simulink model "om1"  (Simulink 7.0)
settings: Solver=ode45  StartTime=0.0  StopTime=10.0  RelTol=1e-3
libraries: cdsFilt x105, cdsIPC x13, cdsEpicsOut x13, cdsMatrix x9, cdsEpicsIn x6, cdsOsc x5, cdsPhase x5, cdsProduct x4, cdsBitwise x4, cdsRms x3, cdsFiltCtrl x2, cdsRfmIO x1
(part 1 of 5)
settings Model: Creator=Rolf  LastModifiedBy=controls  ExtModeAutoUpdateStatusClock=off

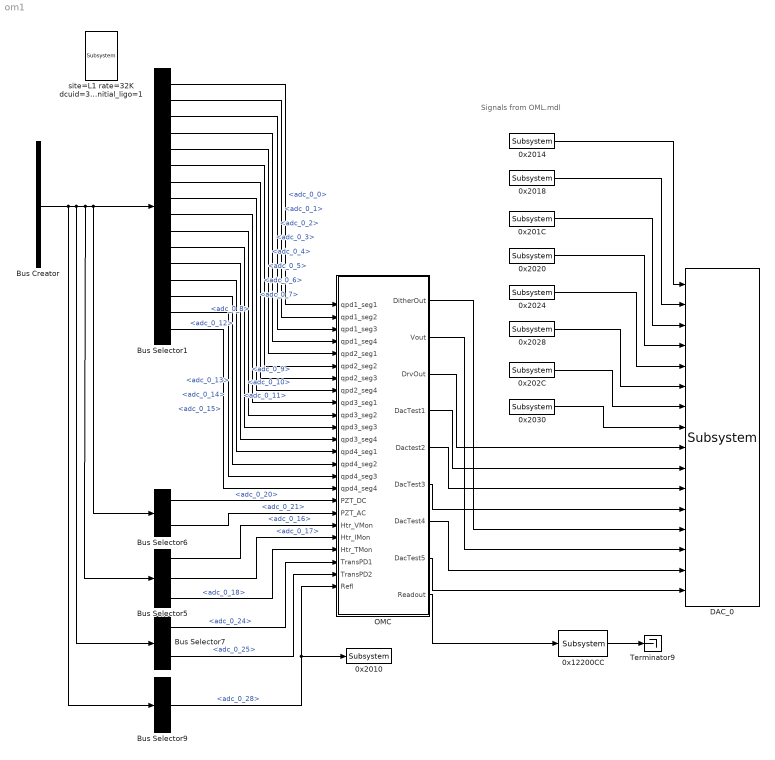
== system om1 ==
  note: Signals from OML.mdl
  0x12200CC : cdsRfmIO/Subsystem  Tag=cdsRfmIO  Description=VMIC5565 Reflective Memory read/write  SystemSampleTime=-1
      settings: AttributesFormatString=%<Tag>
  0x{2010,2014,2018,2020,2024,2028,2030} (7 alike) : cdsIPC/Subsystem  Tag=cdsIPC  Description=Inter-process communication through /rtl_epics_ipc shared memory  SystemSampleTime=-1
      settings: AttributesFormatString=%<Tag>
  0x201C : cdsIPC/Subsystem  Tag=cdsIPC  Description=Inter-process communication through /rtl_epics_ipc shared memory  SystemSampleTime=-1
      settings: AttributesFormatString=%<Tag>
  0x202C : cdsIPC/Subsystem  Tag=cdsIPC  Description=Inter-process communication through /rtl_epics_ipc shared memory  SystemSampleTime=-1
      settings: AttributesFormatString=%<Tag>
  Bus Creator : BusCreator  Tag=adc_0  Description=|  Inputs='adc_0_0','adc_0_1','adc_0_2','adc_0_3','adc_0_4','adc_0_5','adc_0_6','adc_0_7','adc_0_8','adc_0_9','adc_0_10','adc_0_11','adc_0_12','adc_0_13','adc_0_14','adc_0_15','adc_0_16','adc_0_17','adc_0_18','adc_0_19','adc_0_20','adc_0_21','adc_0_22','adc_0_23','adc_0_24','adc_0_25','adc_0_26','adc_0_27','adc_0_28','adc_0_29','adc_0_30','adc_0_31'
      | PCI66-16AI64SSA            
      | 40Vp-p, 16-bit, 610uV/count
      | card_num=1
      settings: AttributesFormatString=%<Description>\n%<Tag>
  Bus Selector1 : BusSelector  OutputSignals=adc_0_0,adc_0_1,adc_0_2,adc_0_3,adc_0_4,adc_0_5,adc_0_6,adc_0_7,adc_0_8,adc_0_9,adc_0_10,adc_0_11,adc_0_12,adc_0_13,adc_0_14,adc_0_15
  Bus Selector5 : BusSelector  OutputSignals=adc_0_16,adc_0_17,adc_0_18
  Bus Selector6 : BusSelector  OutputSignals=adc_0_20,adc_0_21
  Bus Selector7 : BusSelector  OutputSignals=adc_0_24,adc_0_25
  Bus Selector9 : BusSelector  OutputSignals=adc_0_28
  DAC_0 : dac/Subsystem  Description=|  SystemSampleTime=-1
      | PCI66-16AO16
      | 20Vp-p, 16-bit, 305uV/count
      settings: AttributesFormatString=%<Description>
  OMC : Subsystem  Tag=top_names
      settings: AttributesFormatString=%<Tag>
  Terminator9 : Terminator
  site=L1 rate=32K dcuid=30 gds_node_id=4 no_sync=1 compat_initial_ligo=1 : cdsParameters/Subsystem  Tag=cdsParameters  SystemSampleTime=-1
      settings: AttributesFormatString=%<Tag>
  wires:
  Bus Creator/1 -> Bus Selector5/1, Bus Selector1/1, Bus Selector6/1, Bus Selector7/1, Bus Selector9/1
  Bus Selector6/1 -> OMC/17(PZT_DC)  "<adc_0_20>"
  Bus Selector6/2 -> OMC/18(PZT_AC)  "<adc_0_21>"
  Bus Selector7/1 -> OMC/22(TransPD1)  "<adc_0_24>"
  Bus Selector7/2 -> OMC/23(TransPD2)  "<adc_0_25>"
  Bus Selector9/1 -> OMC/24(Refl), 0x2010/1  "<adc_0_28>"
  Bus Selector5/1 -> OMC/19(Htr_VMon)  "<adc_0_16>"
  Bus Selector5/2 -> OMC/20(Htr_IMon)  "<adc_0_17>"
  Bus Selector5/3 -> OMC/21(Htr_TMon)  "<adc_0_18>"
  Bus Selector1/1 -> OMC/1(qpd1_seg1)  "<adc_0_0>"
  Bus Selector1/2 -> OMC/2(qpd1_seg2)  "<adc_0_1>"
  Bus Selector1/3 -> OMC/3(qpd1_seg3)  "<adc_0_2>"
  Bus Selector1/4 -> OMC/4(qpd1_seg4)  "<adc_0_3>"
  Bus Selector1/9 -> OMC/9(qpd3_seg1)  "<adc_0_8>"
  Bus Selector1/10 -> OMC/10(qpd3_seg2)  "<adc_0_9>"
  Bus Selector1/11 -> OMC/11(qpd3_seg3)  "<adc_0_10>"
  Bus Selector1/12 -> OMC/12(qpd3_seg4)  "<adc_0_11>"
  Bus Selector1/5 -> OMC/5(qpd2_seg1)  "<adc_0_4>"
  Bus Selector1/6 -> OMC/6(qpd2_seg2)  "<adc_0_5>"
  Bus Selector1/7 -> OMC/7(qpd2_seg3)  "<adc_0_6>"
  Bus Selector1/8 -> OMC/8(qpd2_seg4)  "<adc_0_7>"
  Bus Selector1/13 -> OMC/13(qpd4_seg1)  "<adc_0_12>"
  Bus Selector1/14 -> OMC/14(qpd4_seg2)  "<adc_0_13>"
  Bus Selector1/15 -> OMC/15(qpd4_seg3)  "<adc_0_14>"
  Bus Selector1/16 -> OMC/16(qpd4_seg4)  "<adc_0_15>"
  OMC/4(DacTest1) -> DAC_0/10
  OMC/5(Dactest2) -> DAC_0/11
  OMC/6(DacTest3) -> DAC_0/12
  OMC/7(DacTest4) -> DAC_0/15
  OMC/8(DacTest5) -> DAC_0/16
  OMC/3(DrvOut) -> DAC_0/9
  OMC/1(DitherOut) -> DAC_0/13
  OMC/2(Vout) -> DAC_0/14
  0x2014/1 -> DAC_0/1
  0x2018/1 -> DAC_0/2
  0x201C/1 -> DAC_0/3
  0x2020/1 -> DAC_0/4
  0x2024/1 -> DAC_0/5
  0x2028/1 -> DAC_0/6
  0x202C/1 -> DAC_0/7
  0x2030/1 -> DAC_0/8
  0x12200CC/1 -> Terminator9/1
  OMC/9(Readout) -> 0x12200CC/1

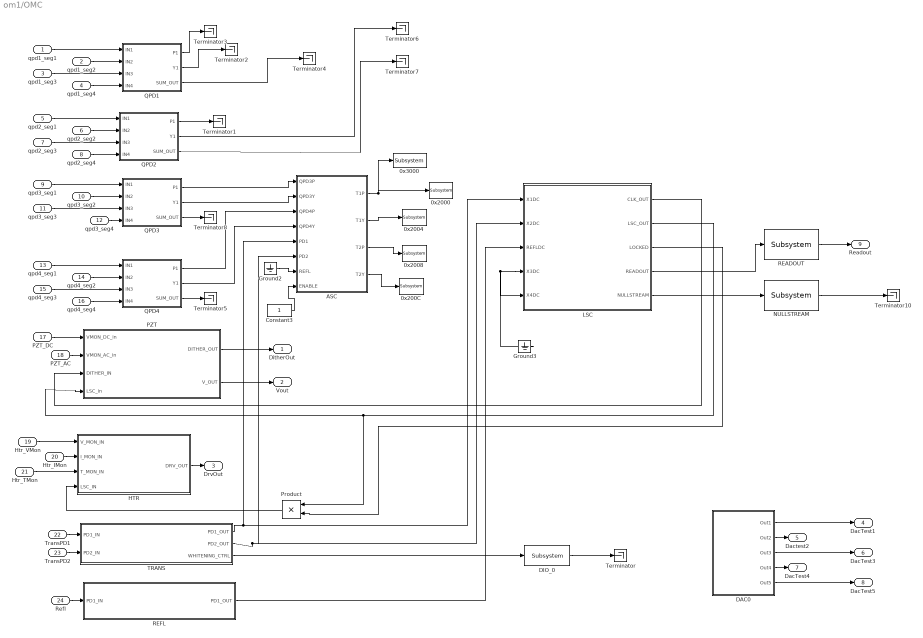
== system om1/OMC ==
  qpd1_seg1 : Inport
  qpd1_seg2 : Inport  Port=2
  qpd1_seg3 : Inport  Port=3
  qpd1_seg4 : Inport  Port=4
  qpd2_seg1 : Inport  Port=5
  qpd2_seg2 : Inport  Port=6
  qpd2_seg3 : Inport  Port=7
  qpd2_seg4 : Inport  Port=8
  qpd3_seg1 : Inport  Port=9
  qpd3_seg2 : Inport  Port=10
  qpd3_seg3 : Inport  Port=11
  qpd3_seg4 : Inport  Port=12
  qpd4_seg1 : Inport  Port=13
  qpd4_seg2 : Inport  Port=14
  qpd4_seg3 : Inport  Port=15
  qpd4_seg4 : Inport  Port=16
  PZT_DC : Inport  Port=17
  PZT_AC : Inport  Port=18
  Htr_VMon : Inport  Port=19
  Htr_IMon : Inport  Port=20
  Htr_TMon : Inport  Port=21
  TransPD1 : Inport  Port=22
  TransPD2 : Inport  Port=23
  Refl : Inport  Port=24
  0x2000 : cdsIPC/Subsystem  Tag=cdsIPC  Description=Inter-process communication through /rtl_epics_ipc shared memory  SystemSampleTime=-1
      settings: AttributesFormatString=%<Tag>
  0x2004 : cdsIPC/Subsystem  Tag=cdsIPC  Description=Inter-process communication through /rtl_epics_ipc shared memory  SystemSampleTime=-1
      settings: AttributesFormatString=%<Tag>
  0x2008 : cdsIPC/Subsystem  Tag=cdsIPC  Description=Inter-process communication through /rtl_epics_ipc shared memory  SystemSampleTime=-1
      settings: AttributesFormatString=%<Tag>
  0x200C : cdsIPC/Subsystem  Tag=cdsIPC  Description=Inter-process communication through /rtl_epics_ipc shared memory  SystemSampleTime=-1
      settings: AttributesFormatString=%<Tag>
  0x3000 : cdsIPCS/Subsystem  Tag=cdsIPCS  SystemSampleTime=-1
      settings: AttributesFormatString=%<Tag>
  ASC : Subsystem
  Constant3 : Constant  OutDataType=sfix(16)  OutScaling=2^0
  DAC0 : Subsystem
  DIO_0 : cdsRio/Subsystem  Tag=cdsRio  Description=PCI IIRO 8 relay output and isolated input module  SystemSampleTime=-1
      settings: AttributesFormatString=%<Tag>
  Ground2 : Ground
  Ground3 : Ground
  HTR : Subsystem
  LSC : Subsystem
  NULLSTREAM : cdsFilt/Subsystem  Tag=cdsFilt  Description=|  SystemSampleTime=-1
      | Purpose:                                                                                                                                                                                                                                  
      | Standard CDS IIR filter module.                                                                                                                                                                                                           
      |                                                                                                                                                                                                                                           
      | Operation:                                                                                                                                                                                                                                
      | Consists of 10 second order section IIR filters, plus a ramped gain stage. In FE code, also provides pre-defined test points and excitation channel inputs. The filter coefficients are defined in the LIGO system using the 'foton' tool.
      |                                                                                                                                                                                                                                           
      | Usage:                                                                                                                                                                                                                                    
      | Name the part with the desired filter module name.
      settings: AttributesFormatString=%<Tag>
  PZT : Subsystem
  Product : Product  Orientation=left  OutDataType=sfix(16)  OutScaling=2^0  RndMeth=Zero
  QPD1 : Subsystem  Description=QPD monitors
      settings: AttributesFormatString=%<Description>
  QPD2 : Subsystem  Description=QPD monitors
      settings: AttributesFormatString=%<Description>
  QPD3 : Subsystem  Description=QPD monitors
      settings: AttributesFormatString=%<Description>
  QPD4 : Subsystem  Description=QPD monitors
      settings: AttributesFormatString=%<Description>
  READOUT : cdsFilt/Subsystem  Tag=cdsFilt  Description=|  SystemSampleTime=-1
      | Purpose:                                                                                                                                                                                                                                  
      | Standard CDS IIR filter module.                                                                                                                                                                                                           
      |                                                                                                                                                                                                                                           
      | Operation:                                                                                                                                                                                                                                
      | Consists of 10 second order section IIR filters, plus a ramped gain stage. In FE code, also provides pre-defined test points and excitation channel inputs. The filter coefficients are defined in the LIGO system using the 'foton' tool.
      |                                                                                                                                                                                                                                           
      | Usage:                                                                                                                                                                                                                                    
      | Name the part with the desired filter module name.
      settings: AttributesFormatString=%<Tag>
  REFL : Subsystem
  TRANS : Subsystem
  Terminator{,1..8,10} (10 alike) : Terminator
  DitherOut : Outport
  Vout : Outport  Port=2
  DrvOut : Outport  Port=3
  DacTest1 : Outport  Port=4
  Dactest2 : Outport  Port=5
  DacTest3 : Outport  Port=6
  DacTest4 : Outport  Port=7
  DacTest5 : Outport  Port=8
  Readout : Outport  Port=9
  wires:
  TRANS/1(PD1_OUT) -> ASC/5(PD1), LSC/1(X1DC)
  TRANS/2(PD2_OUT) -> ASC/6(PD2), LSC/2(X2DC)
  Ground2/1 -> ASC/7(REFL)
  Ground3/1 -> LSC/5(X4DC), LSC/4(X3DC)
  REFL/1(PD1_OUT) -> LSC/3(REFLDC)
  LSC/1(CLK_OUT) -> PZT/3(DITHER_IN)
  LSC/2(LSC_OUT) -> PZT/4(LSC_in), Product/1
  QPD3/1(P1) -> ASC/1(QPD3P)
  QPD3/2(Y1) -> ASC/2(QPD3Y)
  QPD4/1(P1) -> ASC/3(QPD4P)
  QPD4/2(Y1) -> ASC/4(QPD4Y)
  QPD1/3(SUM_OUT) -> Terminator4/1
  QPD2/2(Y1) -> Terminator6/1
  QPD2/3(SUM_OUT) -> Terminator7/1
  DIO_0/1 -> Terminator/1
  TRANS/3(WHITENING_CTRL) -> DIO_0/1
  Product/1 -> HTR/4(LSC_IN)
  LSC/3(LOCKED) -> Product/2
  LSC/4(READOUT) -> READOUT/1
  READOUT/1 -> Readout/1
  QPD1/1(P1) -> Terminator3/1
  QPD1/2(Y1) -> Terminator2/1
  ASC/1(T1P) -> 0x3000/1, 0x2000/1
  ASC/2(T1Y) -> 0x2004/1
  ASC/3(T2P) -> 0x2008/1
  ASC/4(T2Y) -> 0x200C/1
  QPD4/3(SUM_OUT) -> Terminator5/1
  QPD2/1(P1) -> Terminator1/1
  qpd1_seg1/1 -> QPD1/1(IN1)
  qpd1_seg2/1 -> QPD1/2(IN2)
  qpd1_seg3/1 -> QPD1/3(IN3)
  qpd1_seg4/1 -> QPD1/4(IN4)
  qpd2_seg1/1 -> QPD2/1(IN1)
  qpd2_seg2/1 -> QPD2/2(IN2)
  qpd2_seg3/1 -> QPD2/3(IN3)
  qpd2_seg4/1 -> QPD2/4(IN4)
  qpd3_seg1/1 -> QPD3/1(IN1)
  qpd3_seg2/1 -> QPD3/2(IN2)
  qpd3_seg3/1 -> QPD3/3(IN3)
  qpd3_seg4/1 -> QPD3/4(IN4)
  qpd4_seg1/1 -> QPD4/1(IN1)
  qpd4_seg2/1 -> QPD4/2(IN2)
  qpd4_seg3/1 -> QPD4/3(IN3)
  qpd4_seg4/1 -> QPD4/4(IN4)
  PZT_DC/1 -> PZT/1(VMON_DC_in)
  PZT/1(DITHER_OUT) -> DitherOut/1
  PZT_AC/1 -> PZT/2(VMON_AC_in)
  PZT/2(V_OUT) -> Vout/1
  Htr_VMon/1 -> HTR/1(V_MON_IN)
  Htr_IMon/1 -> HTR/2(I_MON_IN)
  HTR/1(DRV_OUT) -> DrvOut/1
  Htr_TMon/1 -> HTR/3(T_MON_IN)
  DAC0/1(Out1) -> DacTest1/1
  TransPD1/1 -> TRANS/1(PD1_IN)
  DAC0/2(Out2) -> Dactest2/1
  DAC0/3(Out3) -> DacTest3/1
  TransPD2/1 -> TRANS/2(PD2_IN)
  DAC0/4(Out4) -> DacTest4/1
  DAC0/5(Out5) -> DacTest5/1
  Refl/1 -> REFL/1(PD1_IN)
  NULLSTREAM/1 -> Terminator10/1
  LSC/5(NULLSTREAM) -> NULLSTREAM/1
  Constant3/1 -> ASC/8(ENABLE)
  QPD3/3(SUM_OUT) -> Terminator8/1
